simulink model "figadidio"  (R2015a)
settings: Solver=ode3  StartTime=0.0  StopTime=10.0  FixedStep=1/200  RelTol=1e-3
undefined symbols (not defined in the file): Aref, B, Bref, GammaR, GammaX, i, P
libraries: PoliArd x6
settings Model: ExtModeTrigDuration=2  Creator=User  LastModifiedBy=user
settings OptimizationCC: OptimizeModelRefInitCode=on  LifeSpan=1
settings DebuggingCC: UnderspecifiedInitializationDetection=Classic  MergeDetectMultiDrivingBlocksExec=none
settings HardwareCC: ProdLargestAtomicInteger=Long  ProdLargestAtomicFloat=Double  ProdEndianess=LittleEndian  ProdHWDeviceType=ARM Compatible->ARM Cortex
settings RTWCC: SystemTargetFile=realtime.tlc  GenerateMakefile=off  TemplateMakefile=realtime.tmf  Description=Run on Target Hardware  RTWVerbose=off
settings ERTTargetCC: CombineOutputUpdateFcns=off  ExtModeTransport=3  ExtModeMexFile=ext_serial_win32_comm_rtt  ExtModeMexArgs=0 1 9600  ERTSrcFileBannerTemplate=realtime_code_template.cgt  ERTHdrFileBannerTemplate=realtime_code_template.cgt  ERTDataSrcFileTemplate=realtime_code_template.cgt  ERTDataHdrFileTemplate=realtime_code_template.cgt  ERTCustomFileTemplate=realtime_file_process.tlc

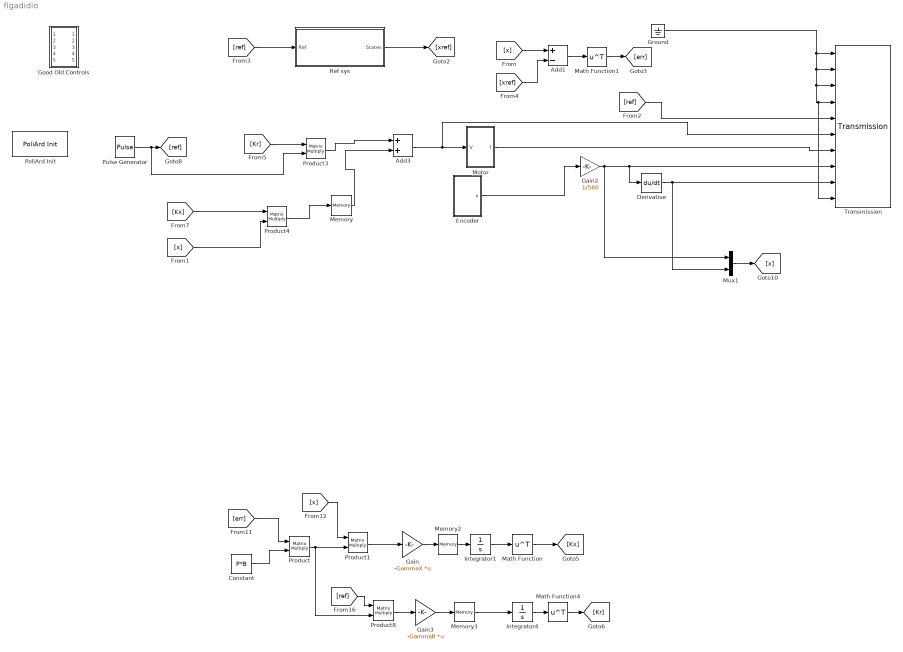
== system figadidio ==
  Add1 : Sum  Inputs=+-
  Add3 : Sum
  Constant : Constant  Value=P*B
  Derivative : Derivative
  "Encoder " : Subsystem
  Gain : Gain  Gain=-GammaX  Multiplication=Matrix(K*u)
  Gain2 : Gain  Gain=1/560
  Gain3 : Gain  Gain=-GammaR  Multiplication=Matrix(K*u)
  Good Old Controls : Subsystem
  Ground : Ground
  Integrator1 : Integrator
  Integrator4 : Integrator
  Math Function : Math  Operator=transpose  SaturateOnIntegerOverflow=on
  Math Function1 : Math  Operator=transpose  SaturateOnIntegerOverflow=on
  Math Function4 : Math  Operator=transpose  SaturateOnIntegerOverflow=on
  Memory : Memory
  Memory2 : Memory
  Memory3 : Memory
  Motor : Subsystem
  Mux1 : Mux  Inputs=2
  PoliArd Init : PoliArd/PoliArd Init
  Product{,1,3..4,8} (5 alike) : Product  Multiplication=Matrix(*)
  Pulse Generator : DiscretePulseGenerator  PulseType=Time based  Amplitude=2  Period=10  PulseWidth=50  PhaseDelay=5
  Ref sys : Subsystem
  Transmission : PoliArd/Transmission  sample_freq=200  sig_to_send=6
  wires:
  Ground/1 -> Transmission/10, Transmission/4, Transmission/3, Transmission/2, Transmission/1
  "Encoder "/1(x) -> Gain2/1
  Derivative/1 -> Mux1/2, Transmission/9
  Gain2/1 -> Mux1/1, Derivative/1, Transmission/8
  Memory/1 -> Add3/2
  Add3/1 -> Transmission/6, Motor/1(V)
  Ref sys/1(States) -> [xref]
  [ref] -> Ref sys/1(Ref)
  [x] -> Add1/1
  [xref] -> Add1/2
  Add1/1 -> Math Function1/1
  Math Function1/1 -> [err]
  Product4/1 -> Memory/1
  [err] -> Product/1
  Constant/1 -> Product/2
  Product/1 -> Product8/2, Product1/2
  [x] -> Product1/1
  Product1/1 -> Gain/1
  Integrator1/1 -> Math Function/1
  [ref] -> Product8/1
  Product8/1 -> Gain3/1
  Integrator4/1 -> Math Function4/1
  Math Function/1 -> [Kx]
  Math Function4/1 -> [Kr]
  Gain/1 -> Memory2/1
  Memory2/1 -> Integrator1/1
  Gain3/1 -> Memory3/1
  Memory3/1 -> Integrator4/1
  Mux1/1 -> [x]
  [Kx] -> Product4/1
  Product3/1 -> Add3/1
  [Kr] -> Product3/1
  [ref] -> Transmission/5
  Motor/1(I) -> Transmission/7
  Pulse Generator/1 -> Product3/2, [ref]
  [x] -> Product4/2

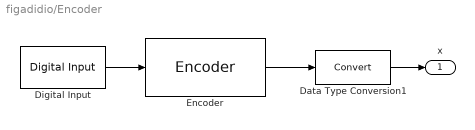
== system figadidio/Encoder  ==
  Data Type Conversion1 : DataTypeConversion
  Digital Input : PoliArd/Digital Input  DI_pin=2  DIsample=1/200
  Encoder : PoliArd/Encoder  EncoderID=1  dt_enc=-1
  x : Outport
  wires:
  Digital Input/1 -> Encoder/1
  Data Type Conversion1/1 -> x/1
  Encoder/1 -> Data Type Conversion1/1

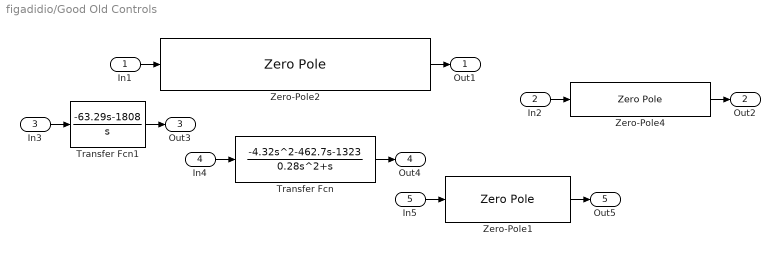
== system figadidio/Good Old Controls ==
  In1 : Inport
  In2 : Inport  Port=2
  In3 : Inport  Port=3
  In4 : Inport  Port=4
  In5 : Inport  Port=5
  Transfer Fcn : TransferFcn  Numerator=[-4.32 -462.7 -1323]  Denominator=[0.28 1 0]
  Transfer Fcn1 : TransferFcn  Numerator=[-63.29 -1808]  Denominator=[1 0]
  Zero-Pole1 : ZeroPole  Zeros=[-5+22i, -5-22i]  Poles=[0, -100]  Gain=-0.03
  Zero-Pole2 : ZeroPole  Zeros=[-79.8,-33.1, -58.4+16.9*i , -58.4-16.9*i]  Poles=[0,-111,-566+45.7*i, -566-45.7*i]  Gain=-4.3815
  Zero-Pole4 : ZeroPole  Zeros=[9.52+3.16i,9.52-3.16i]  Poles=[0,-100]  Gain=-0.016498
  Out1 : Outport
  Out2 : Outport  Port=2
  Out3 : Outport  Port=3
  Out4 : Outport  Port=4
  Out5 : Outport  Port=5
  wires:
  Transfer Fcn1/1 -> Out3/1
  Transfer Fcn/1 -> Out4/1
  In3/1 -> Transfer Fcn1/1
  In2/1 -> Zero-Pole4/1
  In4/1 -> Transfer Fcn/1
  Zero-Pole4/1 -> Out2/1
  In5/1 -> Zero-Pole1/1
  Zero-Pole2/1 -> Out1/1
  Zero-Pole1/1 -> Out5/1
  In1/1 -> Zero-Pole2/1

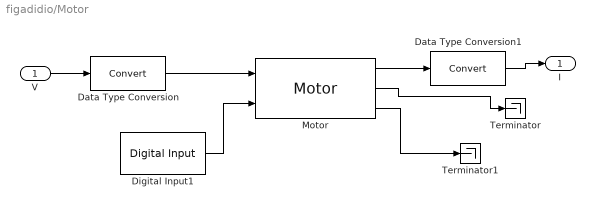
== system figadidio/Motor ==
  V : Inport
  Data Type Conversion : DataTypeConversion
  Data Type Conversion1 : DataTypeConversion
  Digital Input1 : PoliArd/Digital Input  DI_pin=3  DIsample=1/200
  Motor : PoliArd/Motor  MotorID=1  DC_bus_mask=12  dt_mot=1/200
  Terminator : Terminator
  Terminator1 : Terminator
  I : Outport
  wires:
  Data Type Conversion/1 -> Motor/1
  Digital Input1/1 -> Motor/2
  V/1 -> Data Type Conversion/1
  Motor/3 -> Terminator1/1
  Motor/2 -> Terminator/1
  Motor/1 -> Data Type Conversion1/1
  Data Type Conversion1/1 -> I/1

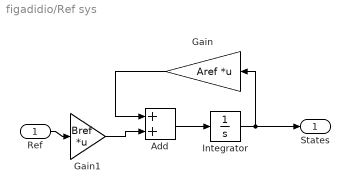
== system figadidio/Ref sys ==
  Ref : Inport
  Add : Sum
  Gain : Gain  Gain=Aref  Multiplication=Matrix(K*u)
  Gain1 : Gain  Gain=Bref  Multiplication=Matrix(K*u)
  Integrator : Integrator
  States : Outport
  wires:
  Gain/1 -> Add/1
  Gain1/1 -> Add/2
  Add/1 -> Integrator/1
  Ref/1 -> Gain1/1
  Integrator/1 -> States/1, Gain/1
